simulink model "problem7"  (R2020b)
settings: Solver=VariableStepAuto  StartTime=0.0  StopTime=10.0  RelTol=1e-3
settings Model: Creator=Sourav Kumar  LastModifiedBy=Sourav Kumar

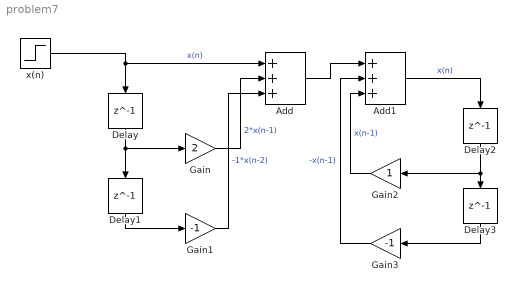
== system problem7 ==
  Add : Sum  Inputs=+++
  Add1 : Sum  Inputs=+++
  Delay{,1..3} (4 alike) : Delay  DelayLength=1
  Gain : Gain  Gain=2
  Gain1 : Gain  Gain=-1
  Gain2 : Gain
  Gain3 : Gain  Gain=-1
  x(n) : Step  SampleTime=0
  wires:
  Delay/1 -> Gain/1, Delay1/1
  Delay2/1 -> Gain2/1, Delay3/1
  Gain2/1 -> Add1/3  "x(n-1)"
  Add1/1 -> Delay2/1  "x(n)"
  Delay3/1 -> Gain3/1
  Gain3/1 -> Add1/2  "-x(n-1)"
  Add/1 -> Add1/1
  Gain1/1 -> Add/3  "-1*x(n-2)"
  Gain/1 -> Add/2  "2*x(n-1)"
  x(n)/1 -> Add/1, Delay/1  "x(n)"
  Delay1/1 -> Gain1/1
